simulink model "cyberAttack"  (R2022b)
settings: Solver=VariableStepAuto  StartTime=0.0  StopTime=10  RelTol=1e-3
values from neighbouring files (symbols this model uses):
  attackTimeDelay = 0.1    [editor.m]
  CC_Kd = 0    [editor.m]
  CC_Ki = 150    [editor.m]
  CC_Kp = 0    [editor.m]
  enableObserver = 1    [editor.m]
  ICapacity_1 = 3    [editor.m]
  ICapacity_2 = 2    [editor.m]
  ILoadFinal = 2    [editor.m]
  ILoadInitial = 3    [editor.m]
  Kd = 4.6e-4    (= 0.00046)    [editor.m]
  Ki = 6.15    [editor.m]
  Kp = 0.1    [editor.m]
  N = 2.56e3    (= 2560)    [editor.m]
  Rij = 0.05    [editor.m]
  Rt = 0.2    [editor.m]
  timeOfAttack = 5    [editor.m]
  tLoadChange = 6    [editor.m]
  Ts = 5e-5    (= 5e-05)    [editor.m]
  Vref = 40    [editor.m]
undefined symbols (not defined in the file or in its folder): Discrete, Time
libraries: fl_lib x27, nesl_utility_internal x15, slpidlib x4, simulink x2, ctrlSharedLib x2, ee_lib x2
(part 2 of 2)

== system cyberAttack/Communication Channel DGU 1 (open to attack)1/Communication Channel ==
  Vt : Inport
  It : Inport  Port=2
  Vout : Inport  Port=3
  tag scope: It_2=global, Vout_2=global, Vt_2=global
  wires:
  Vout/1 -> [Vout_2]
  It/1 -> [It_2]
  Vt/1 -> [Vt_2]

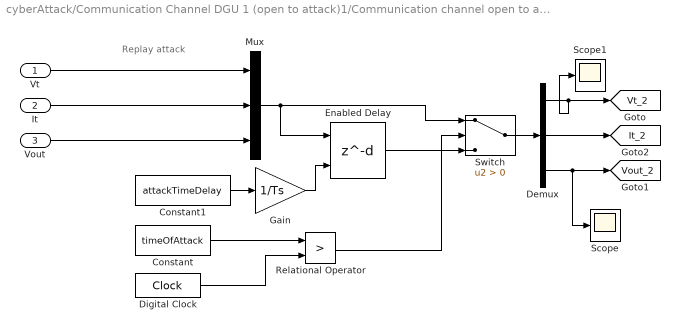
== system cyberAttack/Communication Channel DGU 1 (open to attack)1/Communication channel open to attack ==
  note: Replay attack
  Vt : Inport
  It : Inport  Port=2
  Vout : Inport  Port=3
  Constant : Constant  Value=timeOfAttack
  Constant1 : Constant  Value=attackTimeDelay
  Demux : Demux  Outputs=3
  Digital Clock : DigitalClock
  Enabled Delay : Delay  DelayLengthSource=Input port  DelayLength=attackTimeDelay/Ts  DelayLengthUpperLimit=4000  SampleTime=Ts
      settings: InputPortMap=u0,p1
  Gain : Gain  Gain=1/Ts
  Mux : Mux  Inputs=3
  Relational Operator : RelationalOperator  Operator=>  OutDataTypeStr=boolean  RndMeth=Simplest  InputSameDT=off
  Scope : Scope
  Scope1 : Scope
  Switch : Switch  Criteria=u2 > Threshold  SaturateOnIntegerOverflow=off  InputSameDT=off
  tag scope: It_2=global, Vout_2=global, Vt_2=global
  wires:
  Demux/1 -> Scope1/1, [Vt_2]
  Demux/2 -> [It_2]
  Demux/3 -> Scope/1, [Vout_2]
  Vout/1 -> Mux/3
  It/1 -> Mux/2
  Vt/1 -> Mux/1
  Constant1/1 -> Gain/1
  Constant/1 -> Relational Operator/1
  Switch/1 -> Demux/1
  Mux/1 -> Switch/1, Enabled Delay/1
  Relational Operator/1 -> Switch/2
  Enabled Delay/1 -> Switch/3
  Digital Clock/1 -> Relational Operator/2
  Gain/1 -> Enabled Delay/2

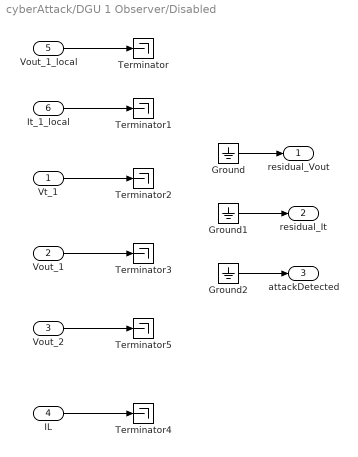
== system cyberAttack/DGU 1 Observer/Disabled ==
  Vt_1 : Inport
  Vout_1 : Inport  Port=2
  Vout_2 : Inport  Port=3
  IL : Inport  Port=4
  Vout_1_local : Inport  Port=5
  It_1_local : Inport  Port=6
  Ground : Ground
  Ground1 : Ground
  Ground2 : Ground
  Terminator{,1..5} (6 alike) : Terminator
  residual_Vout : Outport
  residual_It : Outport  Port=2
  attackDetected : Outport  Port=3
  wires:
  Vt_1/1 -> Terminator2/1
  Vout_1/1 -> Terminator3/1
  Vout_2/1 -> Terminator5/1
  Vout_1_local/1 -> Terminator/1
  It_1_local/1 -> Terminator1/1
  IL/1 -> Terminator4/1
  Ground/1 -> residual_Vout/1
  Ground1/1 -> residual_It/1
  Ground2/1 -> attackDetected/1

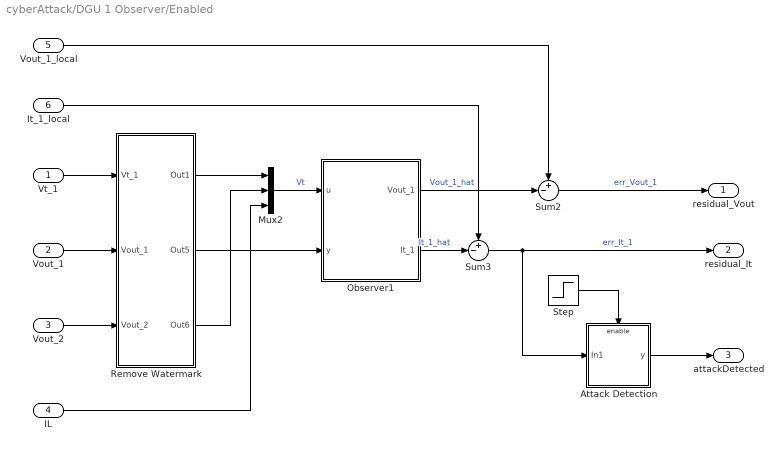
== system cyberAttack/DGU 1 Observer/Enabled ==
  Vt_1 : Inport
  Vout_1 : Inport  Port=2
  Vout_2 : Inport  Port=3
  IL : Inport  Port=4
  Vout_1_local : Inport  Port=5
  It_1_local : Inport  Port=6
  Attack Detection : Subsystem
  Mux2 : Mux  Inputs=3
  Observer1 : Subsystem
  Remove Watermark : Subsystem
  Step : Step  Time=0.3  After=enableObserver  SampleTime=0
  Sum2 : Sum  Inputs=+-|
  Sum3 : Sum  Inputs=+-|
  residual_Vout : Outport
  residual_It : Outport  Port=2
  attackDetected : Outport  Port=3
  wires:
  Mux2/1 -> Observer1/1(u)  "Vt"
  Vt_1/1 -> Remove Watermark/1(Vt_1)
  Vout_1/1 -> Remove Watermark/2(Vout_1)
  Vout_2/1 -> Remove Watermark/3(Vout_2)
  Remove Watermark/3(Out6) -> Mux2/2
  Remove Watermark/2(Out5) -> Observer1/2(y)
  IL/1 -> Mux2/3
  Remove Watermark/1(Out1) -> Mux2/1
  Observer1/1(Vout_1) -> Sum2/2  "Vout_1_hat"
  Sum2/1 -> residual_Vout/1  "err_Vout_1"
  Attack Detection/1(y) -> attackDetected/1
  Observer1/2(It_1) -> Sum3/2  "It_1_hat"
  Sum3/1 -> Attack Detection/1(In1), residual_It/1  "err_It_1"
  Vout_1_local/1 -> Sum2/1
  It_1_local/1 -> Sum3/1
  Step/1 -> Attack Detection/Enable

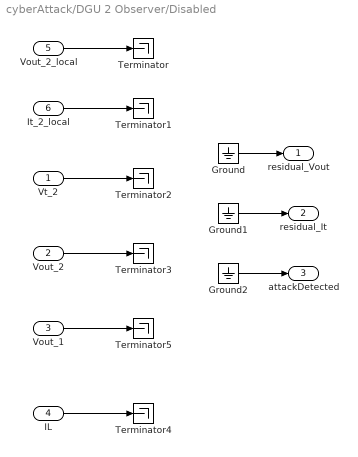
== system cyberAttack/DGU 2 Observer/Disabled ==
  Vt_2 : Inport
  Vout_2 : Inport  Port=2
  Vout_1 : Inport  Port=3
  IL : Inport  Port=4
  Vout_2_local : Inport  Port=5
  It_2_local : Inport  Port=6
  Ground : Ground
  Ground1 : Ground
  Ground2 : Ground
  Terminator{,1..5} (6 alike) : Terminator
  residual_Vout : Outport
  residual_It : Outport  Port=2
  attackDetected : Outport  Port=3
  wires:
  Vt_2/1 -> Terminator2/1
  Vout_2/1 -> Terminator3/1
  Vout_1/1 -> Terminator5/1
  Vout_2_local/1 -> Terminator/1
  It_2_local/1 -> Terminator1/1
  IL/1 -> Terminator4/1
  Ground/1 -> residual_Vout/1
  Ground1/1 -> residual_It/1
  Ground2/1 -> attackDetected/1

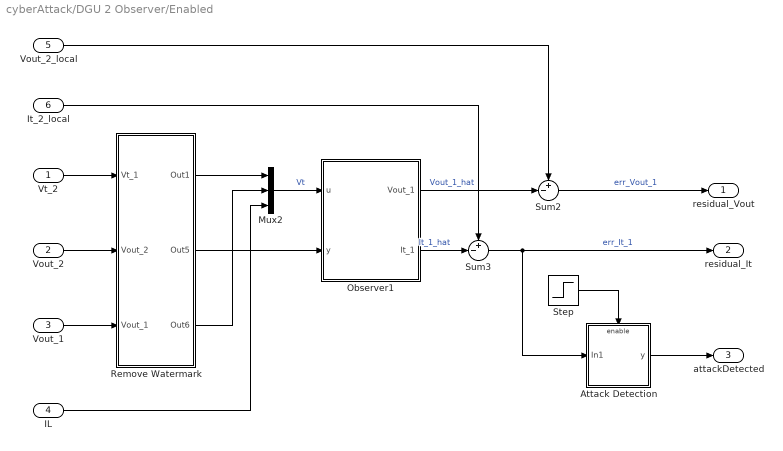
== system cyberAttack/DGU 2 Observer/Enabled ==
  Vt_2 : Inport
  Vout_2 : Inport  Port=2
  Vout_1 : Inport  Port=3
  IL : Inport  Port=4
  Vout_2_local : Inport  Port=5
  It_2_local : Inport  Port=6
  Attack Detection : Subsystem
  Mux2 : Mux  Inputs=3
  Observer1 : Subsystem
  Remove Watermark : Subsystem
  Step : Step  Time=0.3  After=enableObserver  SampleTime=0
  Sum2 : Sum  Inputs=+-|
  Sum3 : Sum  Inputs=+-|
  residual_Vout : Outport
  residual_It : Outport  Port=2
  attackDetected : Outport  Port=3
  wires:
  Mux2/1 -> Observer1/1(u)  "Vt"
  Vt_2/1 -> Remove Watermark/1(Vt_1)
  Vout_2/1 -> Remove Watermark/2(Vout_2)
  Vout_1/1 -> Remove Watermark/3(Vout_1)
  Remove Watermark/3(Out6) -> Mux2/2
  Remove Watermark/2(Out5) -> Observer1/2(y)
  IL/1 -> Mux2/3
  Remove Watermark/1(Out1) -> Mux2/1
  Observer1/1(Vout_1) -> Sum2/2  "Vout_1_hat"
  Sum2/1 -> residual_Vout/1  "err_Vout_1"
  Attack Detection/1(y) -> attackDetected/1
  Observer1/2(It_1) -> Sum3/2  "It_1_hat"
  Sum3/1 -> Attack Detection/1(In1), residual_It/1  "err_It_1"
  Vout_2_local/1 -> Sum2/1
  It_2_local/1 -> Sum3/1
  Step/1 -> Attack Detection/Enable

== system cyberAttack/Voltage controlled DGU 1/PID Controller ==
  Vref : Inport
  Vout : Inport  Port=2
  Delay : Delay  DelayLength=1
  PID Controller : slpidlib/PID Controller  Controller=PID  Form=Parallel  TimeDomain=Discrete-time  UseExternalTs=off  SampleTime=-1  IntegratorMethod=Forward Euler  FilterMethod=Forward Euler  ControllerParametersSource=internal  P=Kp  I=Ki  UseKiTs=off  D=Kd  N=N  UseFilter=on  TunerSelectOption=Transfer Function Based (PID Tuner App)  InitialConditionSource=internal  InitialConditionForIntegrator=0  InitialConditionForFilter=0  DifferentiatorICPrevScaledInput=0  ExternalReset=none  TrackingMode=off  Kt=1  LimitOutput=on  SatLimitsSource=internal  UpperSaturationLimit=0.99  LowerSaturationLimit=0  LinearizeAsGain=on  AntiWindupMode=none  Kb=1  LimitIntegrator=off  UpperIntegratorSaturationLimit=inf  LowerIntegratorSaturationLimit=-inf  POutMin=[]  POutMax=[]  IOutMin=[]  IOutMax=[]  DOutMin=[]  DOutMax=[]  NOutMin=[]  NOutMax=[]  SumOutMin=[]  SumOutMax=[]  SaturationOutMin=[]  SaturationOutMax=[]  PParamMin=[]  PParamMax=[]  IParamMin=[]  IParamMax=[]  DParamMin=[]  DParamMax=[]  NParamMin=[]  NParamMax=[]  KbParamMin=[]  KbParamMax=[]  KtParamMin=[]  KtParamMax=[]  KbOutMin=[]  KbOutMax=[]  KtOutMin=[]  KtOutMax=[]  IntegratorOutMin=[]  IntegratorOutMax=[]  FilterOutMin=[]  FilterOutMax=[]  SumI1OutMin=[]  SumI1OutMax=[]  SumI2OutMin=[]  SumI2OutMax=[]  SumI3OutMin=[]  SumI3OutMax=[]  SumI4OutMin=[]  SumI4OutMax=[]  SumDOutMin=[]  SumDOutMax=[]  DifferentiatorOutMin=[]  DifferentiatorOutMax=[]  FilterDiffOutCoefMin=[]  FilterDiffOutCoefMax=[]  ReciprocalOutMin=[]  ReciprocalOutMax=[]  SumDenOutMin=[]  SumDenOutMax=[]  SumNumOutMin=[]  SumNumOutMax=[]  DivideOutMin=[]  DivideOutMax=[]  UdiffTsProdOutMin=[]  UdiffTsProdOutMax=[]  NTsProdOutMin=[]  NTsProdOutMax=[]  UintegralTsProdOutMin=[]  UintegralTsProdOutMax=[]  UngainTsProdOutMin=[]  UngainTsProdOutMax=[]  ClampingZeroOutDataTypeStr=Inherit: Inherit via back propagation  ClampingZeroOutMin=[]  ClampingZeroOutMax=[]  FilterDenConstantOutDataTypeStr=Inherit: Inherit via back propagation  FilterDenConstantOutMin=[]  FilterDenConstantOutMax=[]  PCopyOutDataTypeStr=Inherit: Inherit via back propagation  PCopyOutMin=[]  PCopyOutMax=[]  NCopyOutDataTypeStr=Inherit: Inherit via back propagation  NCopyOutMin=[]  NCopyOutMax=[]  IntegratorContinuousStateAttributes=''  IntegratorStateMustResolveToSignalObject=off  IntegratorRTWStateStorageClass=Auto  FilterContinuousStateAttributes=''  FilterStateMustResolveToSignalObject=off  FilterRTWStateStorageClass=Auto  ParallelPVariant=InternalParameters  IdealPVariant=Disabled  IVariant=InternalParameters  DVariant=InternalParameters  IntegratorVariant=Discrete  SatVariant=Enabled  AWVariant=Passthrough  PCopyVariant=Disabled  TRVariant=Disabled  FdbkBlocksVariant=Forward  IdealPFdbkVariant=Disabled  SatFdbkVariant=Disabled  DerivativeFilterVariant=ForwardEulerFilter  NVariant=InternalParameters  NCopyVariant=Disabled  FilterICVariant=InternalICsFilter  IntegratorICVariant=InternalICs  ExternalResetVariant=Disabled  TRSumVariant=Passthrough  SumFdbkVariant=Disabled  SumVariant=Sum_PID  TsampFilterVariant=InternalTs  TsampNgainVariant=Passthrough  TsampIntegralVariant=Passthrough  ExternalSaturationOutDataTypeStr=Inherit: Same as second input
  Sum : Sum  Inputs=|+-
  G : Outport
  wires:
  Vref/1 -> Sum/1
  Vout/1 -> Sum/2
  PID Controller/1 -> Delay/1
  Sum/1 -> PID Controller/1
  Delay/1 -> G/1

== system cyberAttack/Voltage controlled DGU 1/Sensing Vin ==
  PS-Simulink Converter4 : nesl_utility_internal/PS-Simulink Converter  PhysicalDomain=network_engine_domain  SubClassName=ps_output  LeftPortType=input  RightPortType=output  PseudoPeriodic=off  Frequencies=[]  VectorFormat=1-D array  Unit=V  AffineConversion=off
  Voltage Sensor : fl_lib/Electrical/Electrical Sensors/Voltage Sensor
  + : PMIOPort  Side=Left
  - : PMIOPort  Port=2  Side=Right
  tag scope: Vin=global
  wires:
  PS-Simulink Converter4/1 -> [Vin]
  connections:
  PS-Simulink Converter4/LConn1 -- Voltage Sensor/RConn1
  Voltage Sensor/RConn2 -- -/RConn1
  Voltage Sensor/LConn1 -- +/RConn1

== system cyberAttack/Voltage controlled DGU 1/Sensing I ==
  Current Sensor : fl_lib/Electrical/Electrical Sensors/Current Sensor
  PS-Simulink Converter3 : nesl_utility_internal/PS-Simulink Converter  PhysicalDomain=network_engine_domain  SubClassName=ps_output  LeftPortType=input  RightPortType=output  PseudoPeriodic=off  Frequencies=[]  VectorFormat=1-D array  Unit=A  AffineConversion=off
  + : PMIOPort  Side=Left
  - : PMIOPort  Port=2  Side=Right
  Iout : Outport
  wires:
  PS-Simulink Converter3/1 -> Iout/1
  connections:
  Current Sensor/RConn2 -- -/RConn1
  Current Sensor/LConn1 -- +/RConn1
  Current Sensor/RConn1 -- PS-Simulink Converter3/LConn1

== system cyberAttack/Voltage controlled DGU 1/Sensing I1 ==
  Current Sensor : fl_lib/Electrical/Electrical Sensors/Current Sensor
  PS-Simulink Converter3 : nesl_utility_internal/PS-Simulink Converter  PhysicalDomain=network_engine_domain  SubClassName=ps_output  LeftPortType=input  RightPortType=output  PseudoPeriodic=off  Frequencies=[]  VectorFormat=1-D array  Unit=A  AffineConversion=off
  + : PMIOPort  Side=Left
  - : PMIOPort  Port=2  Side=Right
  Iout : Outport
  wires:
  PS-Simulink Converter3/1 -> Iout/1
  connections:
  Current Sensor/RConn2 -- -/RConn1
  Current Sensor/LConn1 -- +/RConn1
  Current Sensor/RConn1 -- PS-Simulink Converter3/LConn1

== system cyberAttack/Voltage controlled DGU 1/Voltage Sensing ==
  PS-Simulink Converter4 : nesl_utility_internal/PS-Simulink Converter  PhysicalDomain=network_engine_domain  SubClassName=ps_output  LeftPortType=input  RightPortType=output  PseudoPeriodic=off  Frequencies=[]  VectorFormat=1-D array  Unit=V  AffineConversion=off
  Voltage Sensor : fl_lib/Electrical/Electrical Sensors/Voltage Sensor
  + : PMIOPort  Side=Left
  - : PMIOPort  Port=2  Side=Right
  Out1 : Outport
  wires:
  PS-Simulink Converter4/1 -> Out1/1
  connections:
  Voltage Sensor/LConn1 -- +/RConn1
  Voltage Sensor/RConn2 -- -/RConn1
  PS-Simulink Converter4/LConn1 -- Voltage Sensor/RConn1

== system cyberAttack/Voltage controlled DGU 1/Voltage Sensing1 ==
  PS-Simulink Converter4 : nesl_utility_internal/PS-Simulink Converter  PhysicalDomain=network_engine_domain  SubClassName=ps_output  LeftPortType=input  RightPortType=output  PseudoPeriodic=off  Frequencies=[]  VectorFormat=1-D array  Unit=V  AffineConversion=off
  Voltage Sensor : fl_lib/Electrical/Electrical Sensors/Voltage Sensor
  + : PMIOPort  Side=Left
  - : PMIOPort  Port=2  Side=Right
  Vout : Outport
  wires:
  PS-Simulink Converter4/1 -> Vout/1
  connections:
  Voltage Sensor/LConn1 -- +/RConn1
  Voltage Sensor/RConn2 -- -/RConn1
  PS-Simulink Converter4/LConn1 -- Voltage Sensor/RConn1

== system cyberAttack/Voltage controlled DGU 2/PID Controller ==
  Vref : Inport
  Vout : Inport  Port=2
  Delay : Delay  DelayLength=1
  PID Controller : slpidlib/PID Controller  Controller=PID  Form=Parallel  TimeDomain=Discrete-time  UseExternalTs=off  SampleTime=-1  IntegratorMethod=Forward Euler  FilterMethod=Forward Euler  ControllerParametersSource=internal  P=Kp  I=Ki  UseKiTs=off  D=Kd  N=N  UseFilter=on  TunerSelectOption=Transfer Function Based (PID Tuner App)  InitialConditionSource=internal  InitialConditionForIntegrator=0  InitialConditionForFilter=0  DifferentiatorICPrevScaledInput=0  ExternalReset=none  TrackingMode=off  Kt=1  LimitOutput=on  SatLimitsSource=internal  UpperSaturationLimit=0.99  LowerSaturationLimit=0  LinearizeAsGain=on  AntiWindupMode=none  Kb=1  LimitIntegrator=off  UpperIntegratorSaturationLimit=inf  LowerIntegratorSaturationLimit=-inf  POutMin=[]  POutMax=[]  IOutMin=[]  IOutMax=[]  DOutMin=[]  DOutMax=[]  NOutMin=[]  NOutMax=[]  SumOutMin=[]  SumOutMax=[]  SaturationOutMin=[]  SaturationOutMax=[]  PParamMin=[]  PParamMax=[]  IParamMin=[]  IParamMax=[]  DParamMin=[]  DParamMax=[]  NParamMin=[]  NParamMax=[]  KbParamMin=[]  KbParamMax=[]  KtParamMin=[]  KtParamMax=[]  KbOutMin=[]  KbOutMax=[]  KtOutMin=[]  KtOutMax=[]  IntegratorOutMin=[]  IntegratorOutMax=[]  FilterOutMin=[]  FilterOutMax=[]  SumI1OutMin=[]  SumI1OutMax=[]  SumI2OutMin=[]  SumI2OutMax=[]  SumI3OutMin=[]  SumI3OutMax=[]  SumI4OutMin=[]  SumI4OutMax=[]  SumDOutMin=[]  SumDOutMax=[]  DifferentiatorOutMin=[]  DifferentiatorOutMax=[]  FilterDiffOutCoefMin=[]  FilterDiffOutCoefMax=[]  ReciprocalOutMin=[]  ReciprocalOutMax=[]  SumDenOutMin=[]  SumDenOutMax=[]  SumNumOutMin=[]  SumNumOutMax=[]  DivideOutMin=[]  DivideOutMax=[]  UdiffTsProdOutMin=[]  UdiffTsProdOutMax=[]  NTsProdOutMin=[]  NTsProdOutMax=[]  UintegralTsProdOutMin=[]  UintegralTsProdOutMax=[]  UngainTsProdOutMin=[]  UngainTsProdOutMax=[]  ClampingZeroOutDataTypeStr=Inherit: Inherit via back propagation  ClampingZeroOutMin=[]  ClampingZeroOutMax=[]  FilterDenConstantOutDataTypeStr=Inherit: Inherit via back propagation  FilterDenConstantOutMin=[]  FilterDenConstantOutMax=[]  PCopyOutDataTypeStr=Inherit: Inherit via back propagation  PCopyOutMin=[]  PCopyOutMax=[]  NCopyOutDataTypeStr=Inherit: Inherit via back propagation  NCopyOutMin=[]  NCopyOutMax=[]  IntegratorContinuousStateAttributes=''  IntegratorStateMustResolveToSignalObject=off  IntegratorRTWStateStorageClass=Auto  FilterContinuousStateAttributes=''  FilterStateMustResolveToSignalObject=off  FilterRTWStateStorageClass=Auto  ParallelPVariant=InternalParameters  IdealPVariant=Disabled  IVariant=InternalParameters  DVariant=InternalParameters  IntegratorVariant=Discrete  SatVariant=Enabled  AWVariant=Passthrough  PCopyVariant=Disabled  TRVariant=Disabled  FdbkBlocksVariant=Forward  IdealPFdbkVariant=Disabled  SatFdbkVariant=Disabled  DerivativeFilterVariant=ForwardEulerFilter  NVariant=InternalParameters  NCopyVariant=Disabled  FilterICVariant=InternalICsFilter  IntegratorICVariant=InternalICs  ExternalResetVariant=Disabled  TRSumVariant=Passthrough  SumFdbkVariant=Disabled  SumVariant=Sum_PID  TsampFilterVariant=InternalTs  TsampNgainVariant=Passthrough  TsampIntegralVariant=Passthrough  ExternalSaturationOutDataTypeStr=Inherit: Same as second input
  Sum : Sum  Inputs=|+-
  G : Outport
  wires:
  Vref/1 -> Sum/1
  Vout/1 -> Sum/2
  PID Controller/1 -> Delay/1
  Sum/1 -> PID Controller/1
  Delay/1 -> G/1

== system cyberAttack/Voltage controlled DGU 2/Sensing Vin ==
  PS-Simulink Converter4 : nesl_utility_internal/PS-Simulink Converter  PhysicalDomain=network_engine_domain  SubClassName=ps_output  LeftPortType=input  RightPortType=output  PseudoPeriodic=off  Frequencies=[]  VectorFormat=1-D array  Unit=V  AffineConversion=off
  Voltage Sensor : fl_lib/Electrical/Electrical Sensors/Voltage Sensor
  + : PMIOPort  Side=Left
  - : PMIOPort  Port=2  Side=Right
  tag scope: Vin2=global
  wires:
  PS-Simulink Converter4/1 -> [Vin2]
  connections:
  PS-Simulink Converter4/LConn1 -- Voltage Sensor/RConn1
  Voltage Sensor/RConn2 -- -/RConn1
  Voltage Sensor/LConn1 -- +/RConn1

== system cyberAttack/Voltage controlled DGU 2/Sensing I ==
  Current Sensor : fl_lib/Electrical/Electrical Sensors/Current Sensor
  PS-Simulink Converter3 : nesl_utility_internal/PS-Simulink Converter  PhysicalDomain=network_engine_domain  SubClassName=ps_output  LeftPortType=input  RightPortType=output  PseudoPeriodic=off  Frequencies=[]  VectorFormat=1-D array  Unit=A  AffineConversion=off
  + : PMIOPort  Side=Left
  - : PMIOPort  Port=2  Side=Right
  Iout : Outport
  wires:
  PS-Simulink Converter3/1 -> Iout/1
  connections:
  Current Sensor/RConn2 -- -/RConn1
  Current Sensor/LConn1 -- +/RConn1
  Current Sensor/RConn1 -- PS-Simulink Converter3/LConn1

== system cyberAttack/Voltage controlled DGU 2/Sensing I1 ==
  Current Sensor : fl_lib/Electrical/Electrical Sensors/Current Sensor
  PS-Simulink Converter3 : nesl_utility_internal/PS-Simulink Converter  PhysicalDomain=network_engine_domain  SubClassName=ps_output  LeftPortType=input  RightPortType=output  PseudoPeriodic=off  Frequencies=[]  VectorFormat=1-D array  Unit=A  AffineConversion=off
  + : PMIOPort  Side=Left
  - : PMIOPort  Port=2  Side=Right
  Iout : Outport
  wires:
  PS-Simulink Converter3/1 -> Iout/1
  connections:
  Current Sensor/RConn2 -- -/RConn1
  Current Sensor/LConn1 -- +/RConn1
  Current Sensor/RConn1 -- PS-Simulink Converter3/LConn1

== system cyberAttack/Voltage controlled DGU 2/Voltage Sensing ==
  PS-Simulink Converter4 : nesl_utility_internal/PS-Simulink Converter  PhysicalDomain=network_engine_domain  SubClassName=ps_output  LeftPortType=input  RightPortType=output  PseudoPeriodic=off  Frequencies=[]  VectorFormat=1-D array  Unit=V  AffineConversion=off
  Voltage Sensor : fl_lib/Electrical/Electrical Sensors/Voltage Sensor
  + : PMIOPort  Side=Left
  - : PMIOPort  Port=2  Side=Right
  Out1 : Outport
  wires:
  PS-Simulink Converter4/1 -> Out1/1
  connections:
  Voltage Sensor/LConn1 -- +/RConn1
  Voltage Sensor/RConn2 -- -/RConn1
  PS-Simulink Converter4/LConn1 -- Voltage Sensor/RConn1

== system cyberAttack/Voltage controlled DGU 2/Voltage Sensing1 ==
  PS-Simulink Converter4 : nesl_utility_internal/PS-Simulink Converter  PhysicalDomain=network_engine_domain  SubClassName=ps_output  LeftPortType=input  RightPortType=output  PseudoPeriodic=off  Frequencies=[]  VectorFormat=1-D array  Unit=V  AffineConversion=off
  Voltage Sensor : fl_lib/Electrical/Electrical Sensors/Voltage Sensor
  + : PMIOPort  Side=Left
  - : PMIOPort  Port=2  Side=Right
  Vout : Outport
  wires:
  PS-Simulink Converter4/1 -> Vout/1
  connections:
  Voltage Sensor/LConn1 -- +/RConn1
  Voltage Sensor/RConn2 -- -/RConn1
  PS-Simulink Converter4/LConn1 -- Voltage Sensor/RConn1

== system cyberAttack/Add Watermark 1/Enabled/Add Watermark ==
  y : Inport
  Rate Transition : RateTransition  OutPortSampleTime=Ts
  Scope : Scope
  Sum : Sum  Inputs=|++
  Watermark Signal : SignalGenerator  WaveForm=sawtooth  Amplitude=MP_SawtoothAmplitude  Frequency=MP_SawtoothFrequency
  y_ym : Outport
  wm : Outport  Port=2
  wires:
  y/1 -> Sum/1
  Sum/1 -> y_ym/1
  Watermark Signal/1 -> Scope/1, Rate Transition/1
  Rate Transition/1 -> wm/1, Sum/2

== system cyberAttack/Add Watermark 1/Enabled/Add Watermark1 ==
  y : Inport
  Rate Transition : RateTransition  OutPortSampleTime=Ts
  Sum : Sum  Inputs=|++
  Watermark Signal : SignalGenerator  WaveForm=sawtooth  Amplitude=MP_SawtoothAmplitude  Frequency=MP_SawtoothFrequency
  y_ym : Outport
  wm : Outport  Port=2
  wires:
  y/1 -> Sum/1
  Sum/1 -> y_ym/1
  Watermark Signal/1 -> Rate Transition/1
  Rate Transition/1 -> wm/1, Sum/2

== system cyberAttack/Add Watermark 1/Enabled/Add Watermark2 ==
  y : Inport
  Rate Transition : RateTransition  OutPortSampleTime=Ts
  Sum : Sum  Inputs=|++
  Watermark Signal : SignalGenerator  WaveForm=sawtooth  Amplitude=MP_SawtoothAmplitude  Frequency=MP_SawtoothFrequency
  y_ym : Outport
  wm : Outport  Port=2
  wires:
  y/1 -> Sum/1
  Sum/1 -> y_ym/1
  Watermark Signal/1 -> Rate Transition/1
  Rate Transition/1 -> wm/1, Sum/2

== system cyberAttack/Add Watermark 2/Enabled/Add Watermark ==
  y : Inport
  Rate Transition : RateTransition  OutPortSampleTime=Ts
  Scope : Scope
  Sum : Sum  Inputs=|++
  Watermark Signal : SignalGenerator  WaveForm=sawtooth  Amplitude=MP_SawtoothAmplitude  Frequency=MP_SawtoothFrequency
  y_ym : Outport
  wm : Outport  Port=2
  wires:
  y/1 -> Sum/1
  Sum/1 -> y_ym/1
  Watermark Signal/1 -> Scope/1, Rate Transition/1
  Rate Transition/1 -> wm/1, Sum/2

== system cyberAttack/Add Watermark 2/Enabled/Add Watermark1 ==
  y : Inport
  Rate Transition : RateTransition  OutPortSampleTime=Ts
  Sum : Sum  Inputs=|++
  Watermark Signal : SignalGenerator  WaveForm=sawtooth  Amplitude=MP_SawtoothAmplitude  Frequency=MP_SawtoothFrequency
  y_ym : Outport
  wm : Outport  Port=2
  wires:
  y/1 -> Sum/1
  Sum/1 -> y_ym/1
  Watermark Signal/1 -> Rate Transition/1
  Rate Transition/1 -> wm/1, Sum/2

== system cyberAttack/Add Watermark 2/Enabled/Add Watermark2 ==
  y : Inport
  Rate Transition : RateTransition  OutPortSampleTime=Ts
  Sum : Sum  Inputs=|++
  Watermark Signal : SignalGenerator  WaveForm=sawtooth  Amplitude=MP_SawtoothAmplitude  Frequency=MP_SawtoothFrequency
  y_ym : Outport
  wm : Outport  Port=2
  wires:
  y/1 -> Sum/1
  Sum/1 -> y_ym/1
  Watermark Signal/1 -> Rate Transition/1
  Rate Transition/1 -> wm/1, Sum/2

== system cyberAttack/DGU 1 Observer/Enabled/Attack Detection ==
  In1 : Inport
  Enable : EnablePort
  Abs : Abs  SaturateOnIntegerOverflow=off
  Compare To Constant : simulink/Logic and Bit Operations/Compare To Constant  relop=>  const=2  OutDataTypeStr=boolean
  y : Outport
  wires:
  Abs/1 -> Compare To Constant/1
  Compare To Constant/1 -> y/1
  In1/1 -> Abs/1

== system cyberAttack/DGU 1 Observer/Enabled/Observer1 ==
  u : Inport
  y : Inport  Port=2
  Demux : Demux  Outputs=2
  Kalman Filter : ctrlSharedLib/Kalman Filter  TimeDomain=Discrete-Time  UseCurrentEstimator=on  ModelSource=LTI State-Space Variable  ModelSourceVariable=dguPlantD  A=0.95  B=1  C=1  D=0  NumberOfStates=1  NumberOfInputs=1  NumberOfOutputs=1  InitialEstimateSource=Dialog  X0=0  P0=10  UseK=off  UseGH=off  NumberOfProcessNoiseInputs=1  G=1  TimeInvariantG=on  H=0  TimeInvariantH=on  Q=1e-1  TimeInvariantQ=on  R=1e-4  TimeInvariantR=on  N=0  TimeInvariantN=on  AddInputPort=on  AddEnablePort=off  OutputEstimatedY=off  OutputP=off  Ts=-1
  Rate Transition : RateTransition
  Rate Transition1 : RateTransition
  Vout_1 : Outport
  It_1 : Outport  Port=2
  wires:
  Kalman Filter/1 -> Demux/1
  Demux/2 -> It_1/1
  u/1 -> Rate Transition/1
  y/1 -> Rate Transition1/1
  Demux/1 -> Vout_1/1
  Rate Transition/1 -> Kalman Filter/1
  Rate Transition1/1 -> Kalman Filter/2

== system cyberAttack/DGU 1 Observer/Enabled/Remove Watermark ==
  Vt_1 : Inport
  Vout_1 : Inport  Port=2
  Vout_2 : Inport  Port=3
  Sum : Sum  Inputs=-+|
  Sum4 : Sum  Inputs=-+|
  Sum5 : Sum  Inputs=-+|
  Out1 : Outport
  Out5 : Outport  Port=2
  Out6 : Outport  Port=3
  wires:
  [WM_Vt_1] -> Sum/1
  Vt_1/1 -> Sum/2
  Sum/1 -> Out1/1
  [WM_Vout_1] -> Sum4/1
  Vout_2/1 -> Sum5/2
  [WM_Vout_2] -> Sum5/1
  Sum5/1 -> Out6/1
  Sum4/1 -> Out5/1
  Vout_1/1 -> Sum4/2

== system cyberAttack/DGU 2 Observer/Enabled/Attack Detection ==
  In1 : Inport
  Enable : EnablePort
  Abs : Abs  SaturateOnIntegerOverflow=off
  Compare To Constant : simulink/Logic and Bit Operations/Compare To Constant  relop=>  const=2  OutDataTypeStr=boolean
  y : Outport
  wires:
  Abs/1 -> Compare To Constant/1
  Compare To Constant/1 -> y/1
  In1/1 -> Abs/1

== system cyberAttack/DGU 2 Observer/Enabled/Observer1 ==
  u : Inport
  y : Inport  Port=2
  Demux : Demux  Outputs=2
  Kalman Filter : ctrlSharedLib/Kalman Filter  TimeDomain=Discrete-Time  UseCurrentEstimator=on  ModelSource=LTI State-Space Variable  ModelSourceVariable=dguPlantD  A=0.95  B=1  C=1  D=0  NumberOfStates=1  NumberOfInputs=1  NumberOfOutputs=1  InitialEstimateSource=Dialog  X0=0  P0=10  UseK=off  UseGH=off  NumberOfProcessNoiseInputs=1  G=1  TimeInvariantG=on  H=0  TimeInvariantH=on  Q=1e-1  TimeInvariantQ=on  R=1e-4  TimeInvariantR=on  N=0  TimeInvariantN=on  AddInputPort=on  AddEnablePort=off  OutputEstimatedY=off  OutputP=off  Ts=-1
  Rate Transition : RateTransition
  Rate Transition1 : RateTransition
  Vout_1 : Outport
  It_1 : Outport  Port=2
  wires:
  Kalman Filter/1 -> Demux/1
  Demux/2 -> It_1/1
  u/1 -> Rate Transition/1
  y/1 -> Rate Transition1/1
  Demux/1 -> Vout_1/1
  Rate Transition/1 -> Kalman Filter/1
  Rate Transition1/1 -> Kalman Filter/2

== system cyberAttack/DGU 2 Observer/Enabled/Remove Watermark ==
  Vt_1 : Inport
  Vout_2 : Inport  Port=2
  Vout_1 : Inport  Port=3
  Sum : Sum  Inputs=-+|
  Sum4 : Sum  Inputs=-+|
  Sum5 : Sum  Inputs=-+|
  Out1 : Outport
  Out5 : Outport  Port=2
  Out6 : Outport  Port=3
  wires:
  [WM_Vt_1] -> Sum/1
  Vt_1/1 -> Sum/2
  Sum/1 -> Out1/1
  [WM_Vout_2] -> Sum4/1
  Vout_1/1 -> Sum5/2
  [WM_Vout_1] -> Sum5/1
  Sum5/1 -> Out6/1
  Sum4/1 -> Out5/1
  Vout_2/1 -> Sum4/2
